simulink model "Task1_b_1"  (R2024b)
settings: Solver=VariableStepAuto  StartTime=0.0  StopTime=10.0  RelTol=1e-3
settings Model: Creator=max  LastModifiedBy=max

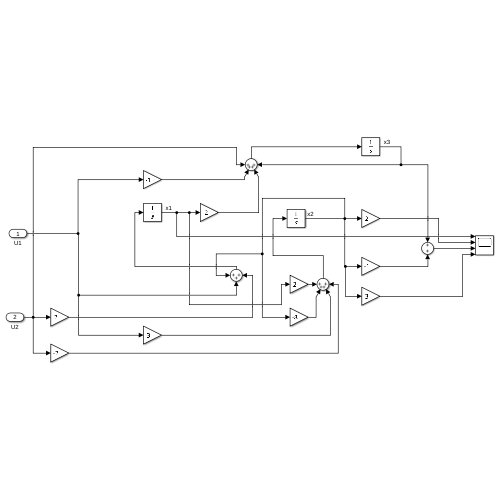
[thumbnail: Simulink's stored preview of the top-level diagram]
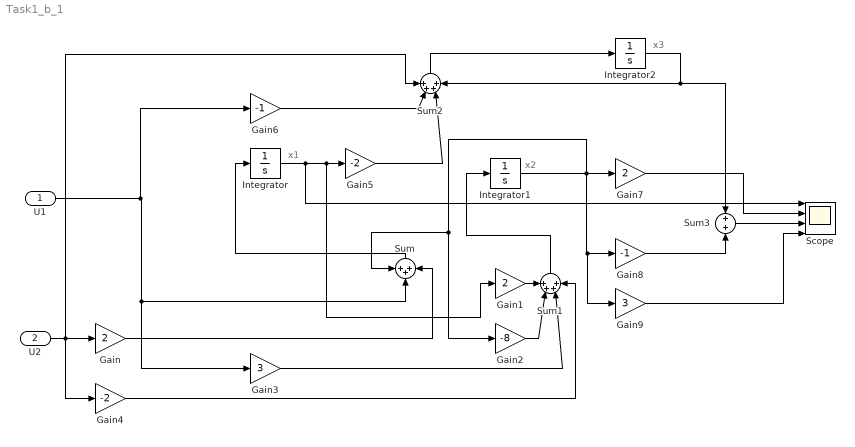
== system Task1_b_1 ==
  note: x3
  note: x2
  note: x1
  U1 : Inport
  U2 : Inport  Port=2
  Gain : Gain  Gain=2
  Gain1 : Gain  Gain=2
  Gain2 : Gain  Gain=-8
  Gain3 : Gain  Gain=3
  Gain4 : Gain  Gain=-2
  Gain5 : Gain  Gain=-2
  Gain6 : Gain  Gain=-1
  Gain7 : Gain  Gain=2
  Gain8 : Gain  Gain=-1
  Gain9 : Gain  Gain=3
  Integrator : Integrator
  Integrator1 : Integrator
  Integrator2 : Integrator
  Scope : Scope  NumInputPorts=4
  Sum : Sum  Inputs=+++
  Sum1 : Sum  Inputs=++++
  Sum2 : Sum  Inputs=++++
  Sum3 : Sum
  wires:
  Integrator1/1 -> Gain9/1, Gain8/1, Gain7/1, Gain2/1, Sum/1
  U1/1 -> Gain6/1, Gain3/1, Sum/2
  U2/1 -> Sum2/1, Gain4/1, Gain/1
  Gain/1 -> Sum/3
  Sum/1 -> Integrator/1
  Gain1/1 -> Sum1/1
  Integrator/1 -> Scope/1, Gain5/1, Gain1/1
  Gain2/1 -> Sum1/2
  Gain3/1 -> Sum1/3
  Gain4/1 -> Sum1/4
  Sum1/1 -> Integrator1/1
  Gain5/1 -> Sum2/3
  Integrator2/1 -> Sum3/1, Sum2/4
  Gain6/1 -> Sum2/2
  Sum2/1 -> Integrator2/1
  Gain7/1 -> Scope/2
  Gain8/1 -> Sum3/2
  Sum3/1 -> Scope/3
  Gain9/1 -> Scope/4
